simulink model "GyroDriftSim"  (R2023a)
settings: Solver=FixedStepAuto  StartTime=0.0  StopTime=simuSteps  FixedStep=1  RelTol=1e-3
undefined symbols (not defined in the file): GyroVal
settings Model: Creator=gusta  LastModifiedBy=gusta

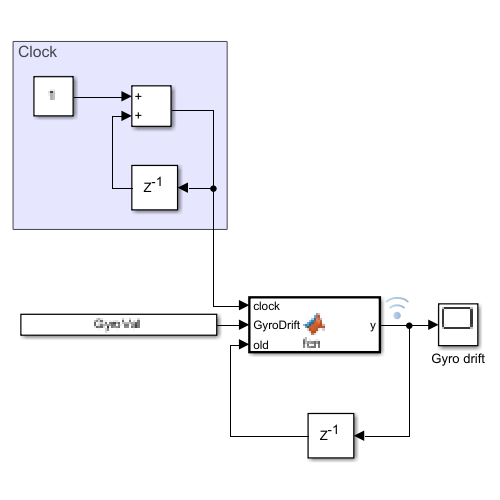
[thumbnail: Simulink's stored preview of the top-level diagram]
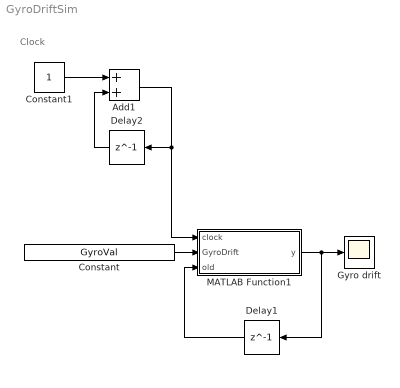
== system GyroDriftSim ==
  note: Clock
  Add1 : Sum
  Constant : Constant  Value=GyroVal
  Constant1 : Constant
  Delay1 : Delay  DelayLength=1
  Delay2 : Delay  DelayLength=1
  Gyro drift : Scope
  MATLAB Function1 : MATLAB Function  TreatAsAtomicUnit=on
  wires:
  Delay1/1 -> MATLAB Function1/3(old)
  Constant/1 -> MATLAB Function1/2(GyroDrift)
  MATLAB Function1/1(y) -> Delay1/1, Gyro drift/1
  Constant1/1 -> Add1/1
  Delay2/1 -> Add1/2
  Add1/1 -> MATLAB Function1/1(clock), Delay2/1

== matlab function GyroDriftSim/MATLAB Function1 ==
  data: clock input; y output; GyroDrift input; old input
function y = fcn(clock,GyroDrift,old)
dt = 0.05;

if(clock == 1)
y = GyroDrift(clock,3)*dt;
else
        y = GyroDrift(clock,3)*dt + old;
end
